simulink library "autolibshared"  (R2019b)
settings: Solver=ode45  StartTime=0.0  StopTime=10.0  RelTol=1e-3  EnableMultiTasking=on
undefined symbols (not defined in the file or in its folder): AccelCycle, aMode, DriveCycle, GearCycle, psi, x_o
libraries: autolibsharedcommon x20, $bdroot x7, autolibutils x2, autolibpowerinfoutils x1
(part 2 of 4)

== system autolibshared/Bicycle Model - Force Input ==
  WhlAngF : Inport  Unit=rad
  FxF : Inport  Port=2  Unit=N
  FxR : Inport  Port=3  Unit=N
  Terminator : Terminator
  Terminator1 : Terminator
  Vehicle Body 3DOF Single Track : $bdroot/Vehicle Body 3DOF Single Track  trackMode=Single (bicycle)  inputMode=External longitudinal forces  frontSteerMode=on  rearSteerMode=off  windMode=off  muMode=off  extFMode=off  extMMode=off  extXo=off  extpsio=off  extxdoto=off  extro=off  extYo=off  extTamb=off  extydoto=off  aMode=aMode  NF=NF  NR=NR  m=m  a=a  b=b  h=h  X_o=X_o  xdot_o=xdot_o  CalphaMode=off  sigmaMode=off  d=0  w=[1.4,1.4]  Cy_f=Cy_f  Cy_r=Cy_r  sigma_f=.1  sigma_r=.1  alpha_f_brk=[-.1 .1]  Cy_f_data=[-9e3 9e3]  alpha_r_brk=[-.1 .1]  Cy_r_data=[-9e3 9e3]  Y_o=Y_o  ydot_o=ydot_o  Izz=Izz  psi_o=psi_o  r_o=r_o  Af=Af  Cd=Cd  Cl=Cl  Cpm=Cpm  beta_w=beta_w  Cs=Cs  Cym=Cym  Pabs=Pabs  Tair=Tair  g=g  mu=mu  xdot_tol=xdot_tol  Fznom=Fznom  Fxtire_sat=Fxtire_sat  Fytire_sat=Fytire_sat  longOff=longOff  latOff=latOff  vertOff=vertOff  wrapAng=off
  Info : Outport  VectorParamsAs1DForOutWhenUnconnected=off
  xdot : Outport  Port=2  VectorParamsAs1DForOutWhenUnconnected=off
  ydot : Outport  Port=3  VectorParamsAs1DForOutWhenUnconnected=off
  psi : Outport  Port=4  VectorParamsAs1DForOutWhenUnconnected=off
  r : Outport  Port=5  VectorParamsAs1DForOutWhenUnconnected=off
  wires:
  Vehicle Body 3DOF Single Track/1 -> Info/1
  Vehicle Body 3DOF Single Track/4 -> psi/1
  WhlAngF/1 -> Vehicle Body 3DOF Single Track/1
  Vehicle Body 3DOF Single Track/2 -> xdot/1
  Vehicle Body 3DOF Single Track/3 -> ydot/1
  Vehicle Body 3DOF Single Track/5 -> r/1
  Vehicle Body 3DOF Single Track/6 -> Terminator1/1
  Vehicle Body 3DOF Single Track/7 -> Terminator/1
  FxF/1 -> Vehicle Body 3DOF Single Track/2
  FxR/1 -> Vehicle Body 3DOF Single Track/3

== system autolibshared/Bicycle Model - Velocity Input ==
  WhlAngF : Inport  Unit=rad
  xdotin : Inport  Port=2  Unit=m/s
  Terminator : Terminator
  Terminator1 : Terminator
  Vehicle Body 3DOF Single Track : $bdroot/Vehicle Body 3DOF Single Track  trackMode=Single (bicycle)  inputMode=External longitudinal velocity  frontSteerMode=on  rearSteerMode=off  windMode=off  muMode=off  extFMode=off  extMMode=off  extXo=off  extpsio=off  extxdoto=off  extro=off  extYo=off  extTamb=off  extydoto=off  aMode=aMode  NF=NF  NR=NR  m=m  a=a  b=b  h=h  X_o=X_o  xdot_o=xdot_o  CalphaMode=off  sigmaMode=off  d=0  w=[1.4,1.4]  Cy_f=Cy_f  Cy_r=Cy_r  sigma_f=.1  sigma_r=.1  alpha_f_brk=[-.1 .1]  Cy_f_data=[-9e3 9e3]  alpha_r_brk=[-.1 .1]  Cy_r_data=[-9e3 9e3]  Y_o=Y_o  ydot_o=ydot_o  Izz=Izz  psi_o=psi_o  r_o=r_o  Af=Af  Cd=Cd  Cl=Cl  Cpm=Cpm  beta_w=beta_w  Cs=Cs  Cym=Cym  Pabs=Pabs  Tair=Tair  g=g  mu=mu  xdot_tol=xdot_tol  Fznom=Fznom  Fxtire_sat=Fxtire_sat  Fytire_sat=Fytire_sat  longOff=longOff  latOff=latOff  vertOff=vertOff  wrapAng=off
  Info : Outport  VectorParamsAs1DForOutWhenUnconnected=off
  xdot : Outport  Port=2  VectorParamsAs1DForOutWhenUnconnected=off
  ydot : Outport  Port=3  VectorParamsAs1DForOutWhenUnconnected=off
  psi : Outport  Port=4  VectorParamsAs1DForOutWhenUnconnected=off
  r : Outport  Port=5  VectorParamsAs1DForOutWhenUnconnected=off
  wires:
  Vehicle Body 3DOF Single Track/7 -> Terminator/1
  xdotin/1 -> Vehicle Body 3DOF Single Track/2
  Vehicle Body 3DOF Single Track/6 -> Terminator1/1
  Vehicle Body 3DOF Single Track/5 -> r/1
  Vehicle Body 3DOF Single Track/3 -> ydot/1
  Vehicle Body 3DOF Single Track/2 -> xdot/1
  WhlAngF/1 -> Vehicle Body 3DOF Single Track/1
  Vehicle Body 3DOF Single Track/4 -> psi/1
  Vehicle Body 3DOF Single Track/1 -> Info/1

== system autolibshared/Drive Cycle Source ==
  Gear : Terminator
  Reference Accel : Terminator
  UnitConversion : UnitConversion
  timing mode : Subsystem  VariantControlMode=Label  Variant=on  LabelModeActiveChoice=1
  Reference Speed : Outport  Unit=m/s  VectorParamsAs1DForOutWhenUnconnected=off
  wires:
  timing mode/3(Gear) -> Gear/1
  UnitConversion/1 -> Reference Speed/1
  timing mode/1(Spd) -> UnitConversion/1
  timing mode/2(Acc) -> Reference Accel/1

== system autolibshared/Longitudinal Driver ==
  VelRef : Inport  Unit=m/s
  VelFdbk : Inport  Port=2  Unit=m/s
  Grade : Inport  Port=3
  ExtGear Ground : Ground
  Gear Terminator : Terminator
  Longitudinal Driver : autolibsharedcommon/Longitudinal Driver  cntrlType=PI  shftType=None  vnom=vnom  Kp=Kp  Ki=Ki  Kaw=Kaw  Kff=Kff  Kg=Kg  tauerr=tauerr  tShift=tShift  tRev=tRev  tPark=tPark  pdlVec=pdlVec  upShftTbl=upShftTbl  dwnShftTbl=dwnShftTbl  GearInit=GearInit  tClutch=tClutch  VehVelVec=VehVelVec  KffVec=KffVec  KiVec=KiVec  KpVec=KpVec  KgVec=KgVec  m=m  Kpt=Kpt  Lvv=L  g=g  UpGearVec=UpGearVec  DownGearVec=DownGearVec  aMode=aMode  errUnit=m/s  aR=aR  bR=bR  cR=cR  tauPt=tauPt
      settings: SourceProductName=Powertrain Blockset  SourceProductBaseCode=PW
  Info : Outport  InitialOutput=0  VectorParamsAs1DForOutWhenUnconnected=off
  AccelCmd : Outport  Port=2  VectorParamsAs1DForOutWhenUnconnected=off
  DecelCmd : Outport  Port=3  VectorParamsAs1DForOutWhenUnconnected=off
  wires:
  VelRef/1 -> Longitudinal Driver/1
  VelFdbk/1 -> Longitudinal Driver/2
  Longitudinal Driver/1 -> Info/1
  Longitudinal Driver/2 -> AccelCmd/1
  Longitudinal Driver/3 -> DecelCmd/1
  Longitudinal Driver/4 -> Gear Terminator/1
  ExtGear Ground/1 -> Longitudinal Driver/4
  Grade/1 -> Longitudinal Driver/3

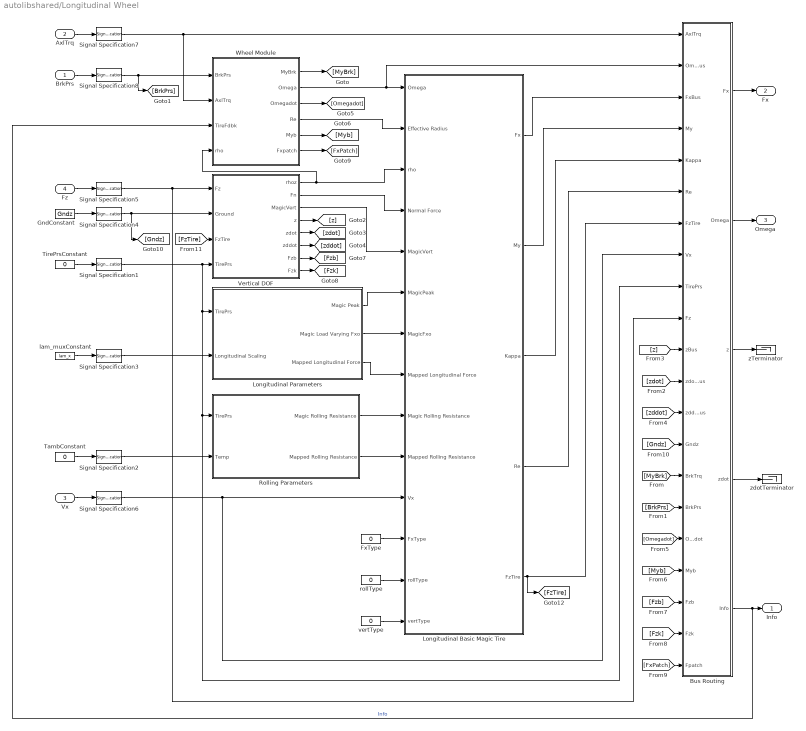
== system autolibshared/Longitudinal Wheel ==
  BrkPrs : Inport
  AxlTrq : Inport  Port=2
  Vx : Inport  Port=3
  Fz : Inport  Port=4
  Bus Routing : Subsystem
  FxType : Constant  Value=0
  GndConstant : Constant  Value=Gndz
  Longitudinal Basic Magic Tire : Subsystem
  Longitudinal Parameters : Subsystem  VariantControlMode=Label  Variant=on  LabelModeActiveChoice=MagicFormulaconstantvalueFx
  Rolling Parameters : Subsystem  VariantControlMode=Label  Variant=on  LabelModeActiveChoice=None
  Signal Specification1 : SignalSpecification  Unit=Pa
  Signal Specification2 : SignalSpecification  Unit=K
  Signal Specification3 : SignalSpecification  Unit=1
  Signal Specification4 : SignalSpecification  Unit=m
  Signal Specification5 : SignalSpecification  Unit=N
  Signal Specification6 : SignalSpecification  Unit=m/s
  Signal Specification7 : SignalSpecification  Unit=N*m
  Signal Specification8 : SignalSpecification  Unit=Pa
  TambConstant : Constant  Value=0
  TirePrsConstant : Constant  Value=0
  Vertical DOF : Subsystem  VariantControlMode=Label  Variant=on  LabelModeActiveChoice=None
  Wheel Module : Subsystem  mask(Wheel Module){aMode=aMode}
  lam_muxConstant : Constant  Value=lam_x
  rollType : Constant  Value=0
  vertType : Constant  Value=0
  zTerminator : Terminator
  zdotTerminator : Terminator
  Info : Outport  VectorParamsAs1DForOutWhenUnconnected=off
  Fx : Outport  Port=2  VectorParamsAs1DForOutWhenUnconnected=off
  Omega : Outport  Port=3  VectorParamsAs1DForOutWhenUnconnected=off
  wires:
  Bus Routing/1(Fx) -> Fx/1
  Bus Routing/5(Info) -> Info/1, Wheel Module/3(TireFdbk)  "Info"
  Bus Routing/2(Omega) -> Omega/1
  Bus Routing/3(z) -> zTerminator/1
  Bus Routing/4(zdot) -> zdotTerminator/1
  TirePrsConstant/1 -> Signal Specification1/1
  Signal Specification2/1 -> Rolling Parameters/2(Temp)
  [BrkPrs] -> Bus Routing/16(BrkPrs)
  Longitudinal Basic Magic Tire/4(Re) -> Bus Routing/6(Re)
  Rolling Parameters/2(Mapped Rolling Resistance) -> Longitudinal Basic Magic Tire/10(Mapped Rolling Resistance)
  Vertical DOF/5(zdot) -> [zdot]
  [zdot] -> Bus Routing/12(zdotBus)
  Longitudinal Basic Magic Tire/2(My) -> Bus Routing/4(My)
  FxType/1 -> Longitudinal Basic Magic Tire/12(FxType)
  Rolling Parameters/1(Magic Rolling Resistance) -> Longitudinal Basic Magic Tire/9(Magic Rolling Resistance)
  Vertical DOF/4(z) -> [z]
  Vertical DOF/3(MagicVert) -> Longitudinal Basic Magic Tire/5(MagicVert)
  Vertical DOF/2(Fn) -> Longitudinal Basic Magic Tire/4(Normal Force)
  rollType/1 -> Longitudinal Basic Magic Tire/13(rollType)
  Longitudinal Parameters/3(Mapped Longitudinal Force) -> Longitudinal Basic Magic Tire/8(Mapped Longitudinal Force)
  Fz/1 -> Signal Specification5/1
  Longitudinal Basic Magic Tire/5(FzTire) -> Bus Routing/7(FzTire), [FzTire]
  Vx/1 -> Signal Specification6/1
  [z] -> Bus Routing/11(zBus)
  Longitudinal Parameters/2(Magic Load Varying Fxo) -> Longitudinal Basic Magic Tire/7(MagicFxo)
  [MyBrk] -> Bus Routing/15(BrkTrq)
  vertType/1 -> Longitudinal Basic Magic Tire/14(vertType)
  AxlTrq/1 -> Signal Specification7/1
  Longitudinal Parameters/1(Magic Peak) -> Longitudinal Basic Magic Tire/6(MagicPeak)
  Vertical DOF/1(rhoz) -> Wheel Module/4(rho), Longitudinal Basic Magic Tire/3(rho)
  Longitudinal Basic Magic Tire/3(Kappa) -> Bus Routing/5(Kappa)
  Longitudinal Basic Magic Tire/1(Fx) -> Bus Routing/3(FxBus)
  Wheel Module/1(MyBrk) -> [MyBrk]
  Wheel Module/2(Omega) -> Bus Routing/2(OmegaBus), Longitudinal Basic Magic Tire/1(Omega)
  Signal Specification1/1 -> Bus Routing/9(TirePrs), Rolling Parameters/1(TirePrs), Longitudinal Parameters/1(TirePrs), Vertical DOF/4(TirePrs)
  Signal Specification3/1 -> Longitudinal Parameters/2(Longitudinal Scaling)
  Signal Specification4/1 -> Vertical DOF/2(Ground), [Gndz]
  Signal Specification5/1 -> Vertical DOF/1(Fz), Bus Routing/10(Fz)
  Signal Specification6/1 -> Longitudinal Basic Magic Tire/11(Vx), Bus Routing/8(Vx)
  Signal Specification7/1 -> Bus Routing/1(AxlTrq), Wheel Module/2(AxlTrq)
  Signal Specification8/1 -> [BrkPrs], Wheel Module/1(BrkPrs)
  lam_muxConstant/1 -> Signal Specification3/1
  TambConstant/1 -> Signal Specification2/1
  Wheel Module/4(Re) -> Longitudinal Basic Magic Tire/2(Effective Radius)
  Vertical DOF/6(zddot) -> [zddot]
  [zddot] -> Bus Routing/13(zddotBus)
  Wheel Module/3(Omegadot) -> [Omegadot]
  [Omegadot] -> Bus Routing/17(Omegadot)
  Wheel Module/5(Myb) -> [Myb]
  [Myb] -> Bus Routing/18(Myb)
  Vertical DOF/8(Fzk) -> [Fzk]
  Vertical DOF/7(Fzb) -> [Fzb]
  [Fzb] -> Bus Routing/19(Fzb)
  [Fzk] -> Bus Routing/20(Fzk)
  Wheel Module/6(Fxpatch) -> [FxPatch]
  [FxPatch] -> Bus Routing/21(Fpatch)
  GndConstant/1 -> Signal Specification4/1
  [Gndz] -> Bus Routing/14(Gndz)
  [FzTire] -> Vertical DOF/3(FzTire)
  BrkPrs/1 -> Signal Specification8/1

== system autolibshared/Vehicle Body 1DOF Longitudinal ==
  FwF : Inport
  FwR : Inport  Port=2
  Grade : Inport  Port=3
  WindX : Inport  Port=4
  AirTempConstant : Constant  Value=T
  FExtConstant : Constant  Value=[0,0,0]
  MExtConstant : Constant  Value=[0,0,0]
  Vehicle Body 1 DOF : autolibsharedcommon/Vehicle Body 1 DOF  VariantControl=SL1dof  m=m  NF=NF  NR=NR  a=a  b=b  h=h  Af=Af  Cd=Cd  Cl=Cl  Cpm=Cpm  T=T  Pabs=Pabs  xdot_o=xdot_o  g=g  aMode=aMode
      settings: SourceProductName=Powertrain Blockset  SourceProductBaseCode=PW
  Info : Outport  VectorParamsAs1DForOutWhenUnconnected=off
  xdot : Outport  Port=2  PortDimensions=1  VectorParamsAs1DForOutWhenUnconnected=off
  FzF : Outport  Port=3  PortDimensions=1  VectorParamsAs1DForOutWhenUnconnected=off
  FzR : Outport  Port=4  PortDimensions=1  VectorParamsAs1DForOutWhenUnconnected=off
  wires:
  FwF/1 -> Vehicle Body 1 DOF/1
  FwR/1 -> Vehicle Body 1 DOF/2
  Grade/1 -> Vehicle Body 1 DOF/3
  WindX/1 -> Vehicle Body 1 DOF/4
  Vehicle Body 1 DOF/1 -> Info/1
  Vehicle Body 1 DOF/2 -> xdot/1
  Vehicle Body 1 DOF/3 -> FzF/1
  Vehicle Body 1 DOF/4 -> FzR/1
  FExtConstant/1 -> Vehicle Body 1 DOF/5
  MExtConstant/1 -> Vehicle Body 1 DOF/6
  AirTempConstant/1 -> Vehicle Body 1 DOF/7

== system autolibshared/Vehicle Body 3DOF Longitudinal ==
  FwF : Inport
  FwR : Inport  Port=2
  Grade : Inport  Port=3
  WindXYZ : Inport  Port=4
  AirTempConstant : Constant  Value=T
  FExtConstant : Constant  Value=[0,0,0]
  MExtConstant : Constant  Value=[0,0,0]
  Vehicle Body 3 DOF Grade Input : autolibsharedcommon/Vehicle Body 3 DOF Grade Input  VariantControl=SL  NF=NF  NR=NR  m=m  a=a  b=b  h=h  Cd=Cd  Af=Af  x_o=x_o  xdot_o=xdot_o  Cl=Cl  z_o=z_o  zdot_o=zdot_o  Iyy=Iyy  Cpm=Cpm  theta_o=theta_o  q_o=q_o  FskF=FskF  dzsF=dzsF  FsbF=FsbF  dzdotsF=dzdotsF  FskR=FskR  dzsR=dzsR  FsbR=FsbR  dzdotsR=dzdotsR  Pabs=Pabs  T=T  g=g  aMode=aMode
      settings: SourceProductName=Powertrain Blockset  SourceProductBaseCode=PW
  Info : Outport  VectorParamsAs1DForOutWhenUnconnected=off
  xdot : Outport  Port=2  VectorParamsAs1DForOutWhenUnconnected=off
  FzF : Outport  Port=3  VectorParamsAs1DForOutWhenUnconnected=off
  FzR : Outport  Port=4  VectorParamsAs1DForOutWhenUnconnected=off
  wires:
  FwF/1 -> Vehicle Body 3 DOF Grade Input/1
  FwR/1 -> Vehicle Body 3 DOF Grade Input/2
  Grade/1 -> Vehicle Body 3 DOF Grade Input/3
  AirTempConstant/1 -> Vehicle Body 3 DOF Grade Input/7
  WindXYZ/1 -> Vehicle Body 3 DOF Grade Input/4
  Vehicle Body 3 DOF Grade Input/3 -> FzF/1
  Vehicle Body 3 DOF Grade Input/4 -> FzR/1
  Vehicle Body 3 DOF Grade Input/1 -> Info/1
  Vehicle Body 3 DOF Grade Input/2 -> xdot/1
  FExtConstant/1 -> Vehicle Body 3 DOF Grade Input/5
  MExtConstant/1 -> Vehicle Body 3 DOF Grade Input/6

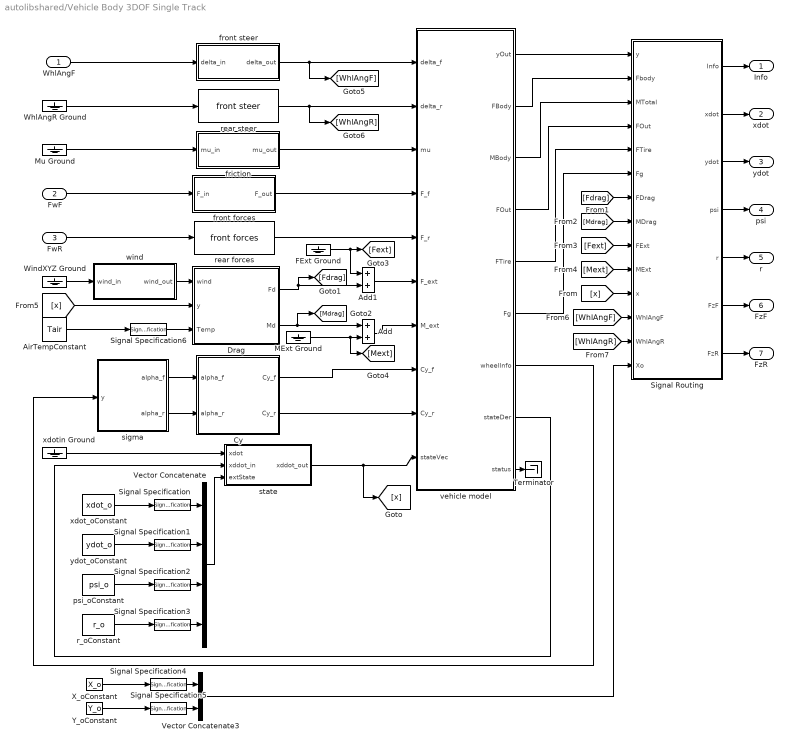
== system autolibshared/Vehicle Body 3DOF Single Track ==
  WhlAngF : Inport
  FwF : Inport  Port=2
  FwR : Inport  Port=3
  Add : Sum
  Add1 : Sum
  AirTempConstant : Constant  Value=Tair
  Cy : Subsystem  VariantControlMode=Label  Variant=on  LabelModeActiveChoice=2
  Drag : Subsystem
  FExt Ground : Ground
  MExt Ground : Ground
  Mu Ground : Ground
  Signal Routing : Subsystem  VariantControlMode=Label  Variant=on  LabelModeActiveChoice=1
  Signal Specification : SignalSpecification  Unit=m/s
  Signal Specification1 : SignalSpecification  Unit=m/s
  Signal Specification2 : SignalSpecification  Unit=rad
  Signal Specification3 : SignalSpecification  Unit=rad/s
  Signal Specification4 : SignalSpecification  Unit=m
  Signal Specification5 : SignalSpecification  Unit=m
  Signal Specification6 : SignalSpecification  Unit=K
  Terminator : Terminator
  Vector Concatenate : Concatenate  NumInputs=4
  Vector Concatenate3 : Concatenate
  WhlAngR Ground : Ground
  WindXYZ Ground : Ground
  X_oConstant : Constant  Value=X_o
  Y_oConstant : Constant  Value=Y_o
  friction : Subsystem  VariantControlMode=Label  Variant=on  LabelModeActiveChoice=2
  front forces : Subsystem  VariantControlMode=Label  Variant=on  LabelModeActiveChoice=4
  front steer : Subsystem  VariantControlMode=Label  Variant=on  LabelModeActiveChoice=3
  psi_oConstant : Constant  Value=psi_o
  r_oConstant : Constant  Value=r_o
  rear forces : $bdroot/Vehicle Body 3DOF Single Track/front forces  SystemSampleTime=-1  LabelModeActiveChoice=4  Latency=0  AutoFrameSizeCalculation=off
  rear steer : $bdroot/Vehicle Body 3DOF Single Track/front steer  SystemSampleTime=-1  LabelModeActiveChoice=2  Latency=0  AutoFrameSizeCalculation=off
  sigma : Subsystem  VariantControlMode=Label  Variant=on  LabelModeActiveChoice=2
  state : Subsystem  VariantControlMode=Label  Variant=on  LabelModeActiveChoice=0
  vehicle model : MATLAB Function  TreatAsAtomicUnit=on
  wind : Subsystem  VariantControlMode=Label  Variant=on  LabelModeActiveChoice=0
  xdot_oConstant : Constant  Value=xdot_o
  xdotin Ground : Ground
  ydot_oConstant : Constant  Value=ydot_o
  Info : Outport  VectorParamsAs1DForOutWhenUnconnected=off
  xdot : Outport  Port=2  VectorParamsAs1DForOutWhenUnconnected=off
  ydot : Outport  Port=3  VectorParamsAs1DForOutWhenUnconnected=off
  psi : Outport  Port=4  VectorParamsAs1DForOutWhenUnconnected=off
  r : Outport  Port=5  VectorParamsAs1DForOutWhenUnconnected=off
  FzF : Outport  Port=6  VectorParamsAs1DForOutWhenUnconnected=off
  FzR : Outport  Port=7  VectorParamsAs1DForOutWhenUnconnected=off
  wires:
  Add1/1 -> vehicle model/6(F_ext)
  Add/1 -> vehicle model/7(M_ext)
  vehicle model/3(MBody) -> Signal Routing/3(MTotal)
  vehicle model/2(FBody) -> Signal Routing/2(Fbody)
  [Mext] -> Signal Routing/10(MExt)
  [Mdrag] -> Signal Routing/8(MDrag)
  [Fdrag] -> Signal Routing/7(FDrag)
  [Fext] -> Signal Routing/9(FExt)
  vehicle model/6(Fg) -> Signal Routing/6(Fg)
  vehicle model/5(FTire) -> Signal Routing/5(FTire)
  vehicle model/9(status) -> Terminator/1
  [x] -> Signal Routing/11(x)
  state/1(xddot_out) -> vehicle model/10(stateVec), [x]
  vehicle model/4(FOut) -> Signal Routing/4(FOut)
  Signal Routing/2(xdot) -> xdot/1
  Signal Routing/7(FzR) -> FzR/1
  Signal Routing/6(FzF) -> FzF/1
  Signal Routing/5(r) -> r/1
  Signal Routing/3(ydot) -> ydot/1
  vehicle model/1(yOut) -> Signal Routing/1(y)
  vehicle model/8(stateDer) -> state/2(xddot_in)
  friction/1(mu_out) -> vehicle model/3(mu)
  Cy/1(Cy_f) -> vehicle model/8(Cy_f)
  Cy/2(Cy_r) -> vehicle model/9(Cy_r)
  front steer/1(delta_out) -> [WhlAngF], vehicle model/1(delta_f)
  rear steer/1 -> [WhlAngR], vehicle model/2(delta_r)
  sigma/1(alpha_f) -> Cy/1(alpha_f)
  sigma/2(alpha_r) -> Cy/2(alpha_r)
  Signal Routing/1(Info) -> Info/1
  vehicle model/7(wheelInfo) -> sigma/1(y)
  front forces/1(F_out) -> vehicle model/4(F_f)
  rear forces/1 -> vehicle model/5(F_r)
  Drag/2(Md) -> [Mdrag], Add/1
  wind/1(wind_out) -> Drag/1(wind)
  Drag/1(Fd) -> Add1/2, [Fdrag]
  WindXYZ Ground/1 -> wind/1(wind_in)
  [x] -> Drag/2(y)
  WhlAngF/1 -> front steer/1(delta_in)
  WhlAngR Ground/1 -> rear steer/1
  Mu Ground/1 -> friction/1(mu_in)
  Signal Routing/4(psi) -> psi/1
  [WhlAngF] -> Signal Routing/12(WhlAngF)
  [WhlAngR] -> Signal Routing/13(WhlAngR)
  Vector Concatenate/1 -> state/3(extState)
  xdot_oConstant/1 -> Signal Specification/1
  Signal Specification/1 -> Vector Concatenate/1
  ydot_oConstant/1 -> Signal Specification1/1
  Signal Specification1/1 -> Vector Concatenate/2
  r_oConstant/1 -> Signal Specification3/1
  psi_oConstant/1 -> Signal Specification2/1
  Signal Specification3/1 -> Vector Concatenate/4
  Signal Specification2/1 -> Vector Concatenate/3
  Vector Concatenate3/1 -> Signal Routing/14(Xo)
  X_oConstant/1 -> Signal Specification4/1
  Signal Specification4/1 -> Vector Concatenate3/1
  Y_oConstant/1 -> Signal Specification5/1
  Signal Specification5/1 -> Vector Concatenate3/2
  Signal Specification6/1 -> Drag/3(Temp)
  AirTempConstant/1 -> Signal Specification6/1
  xdotin Ground/1 -> state/1(xdot)
  FwF/1 -> front forces/1(F_in)
  FwR/1 -> rear forces/1
  MExt Ground/1 -> [Mext], Add/2
  FExt Ground/1 -> Add1/1, [Fext]

== system autolibshared/Vehicle Body Total Road Load ==
  ForceTot : Inport
  Grade : Inport  Port=2
  Vehicle Body Total Road Load : autolibsharedcommon/Vehicle Body Total Road Load  VariantControl=SL1dof  m=m  a=a  b=b  c=c  xdot_o=xdot_o  g=g  x_o=x_o  aMode=aMode
      settings: SourceProductName=Powertrain Blockset  SourceProductBaseCode=PW
  Info : Outport  VectorParamsAs1DForOutWhenUnconnected=off
  xdot : Outport  Port=2  VectorParamsAs1DForOutWhenUnconnected=off
  wires:
  Grade/1 -> Vehicle Body Total Road Load/2
  ForceTot/1 -> Vehicle Body Total Road Load/1
  Vehicle Body Total Road Load/1 -> Info/1
  Vehicle Body Total Road Load/2 -> xdot/1

== system autolibshared/Drive Cycle Source/timing mode ==
  note: 1) Add Subsystem or Model blocks as valid variant choices.
      | 2) You cannot connect blocks at this level. At simulation, connectivity is automatically
      | determined, based on the active variant and port name matching.
  Continuous : Subsystem  VariantControl=1
  Discrete : Subsystem  VariantControl=2
  Spd : Outport  VectorParamsAs1DForOutWhenUnconnected=off
  Acc : Outport  Port=2  VectorParamsAs1DForOutWhenUnconnected=off
  Gear : Outport  Port=3  VectorParamsAs1DForOutWhenUnconnected=off

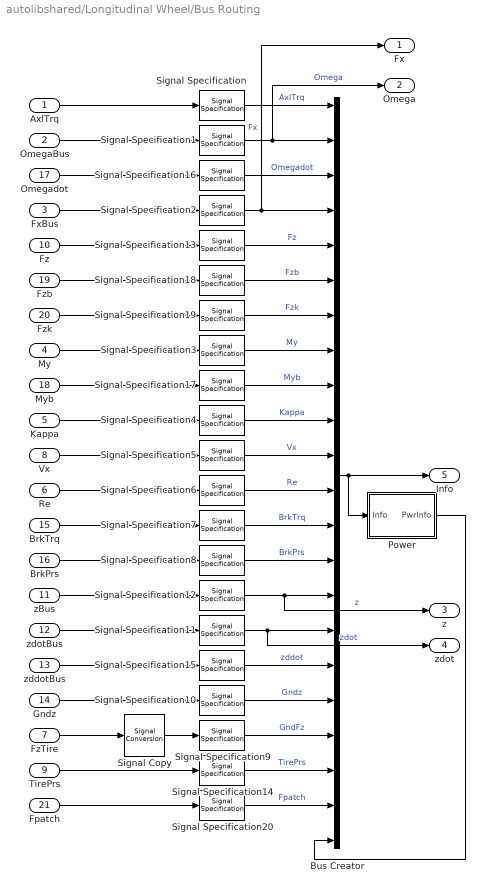
== system autolibshared/Longitudinal Wheel/Bus Routing ==
  AxlTrq : Inport
  OmegaBus : Inport  Port=2
  FxBus : Inport  Port=3
  My : Inport  Port=4
  Kappa : Inport  Port=5
  Re : Inport  Port=6
  FzTire : Inport  Port=7
  Vx : Inport  Port=8
  TirePrs : Inport  Port=9
  Fz : Inport  Port=10
  zBus : Inport  Port=11
  zdotBus : Inport  Port=12
  zddotBus : Inport  Port=13
  Gndz : Inport  Port=14
  BrkTrq : Inport  Port=15
  BrkPrs : Inport  Port=16
  Omegadot : Inport  Port=17
  Myb : Inport  Port=18
  Fzb : Inport  Port=19
  Fzk : Inport  Port=20
  Fpatch : Inport  Port=21
  Bus Creator : BusCreator  Inputs=22
  Power : Subsystem
  Signal Copy : SignalConversion  OverrideOpt=off
  Signal Specification{,3,7,17} (4 alike) : SignalSpecification  Unit=N*m
  Signal Specification1 : SignalSpecification  Unit=rad/s
  Signal Specification10 : SignalSpecification  Unit=m
  Signal Specification11 : SignalSpecification  Unit=m/s
  Signal Specification12 : SignalSpecification  Unit=m
  Signal Specification{2,9,13,18..20} (6 alike) : SignalSpecification  Unit=N
  Signal Specification14 : SignalSpecification  Unit=Pa
  Signal Specification15 : SignalSpecification  Unit=m/s^2
  Signal Specification16 : SignalSpecification  Unit=rad/s^2
  Signal Specification4 : SignalSpecification  Unit=1
  Signal Specification5 : SignalSpecification  Unit=m/s
  Signal Specification6 : SignalSpecification  Unit=m
  Signal Specification8 : SignalSpecification  Unit=Pa
  Fx : Outport  Unit=N  VectorParamsAs1DForOutWhenUnconnected=off
  Omega : Outport  Port=2  Unit=rad/s  VectorParamsAs1DForOutWhenUnconnected=off
  z : Outport  Port=3  Unit=m  VectorParamsAs1DForOutWhenUnconnected=off
  zdot : Outport  Port=4  Unit=m/s  VectorParamsAs1DForOutWhenUnconnected=off
  Info : Outport  Port=5  VectorParamsAs1DForOutWhenUnconnected=off
  wires:
  Signal Specification14/1 -> Bus Creator/20  "TirePrs"
  TirePrs/1 -> Signal Specification14/1
  Re/1 -> Signal Specification6/1
  Fz/1 -> Signal Specification13/1
  Signal Specification13/1 -> Bus Creator/5  "Fz"
  Signal Specification12/1 -> z/1, Bus Creator/15  "z"
  Signal Specification11/1 -> zdot/1, Bus Creator/16  "zdot"
  zdotBus/1 -> Signal Specification11/1
  FzTire/1 -> Signal Copy/1
  Signal Specification9/1 -> Bus Creator/19  "GndFz"
  zBus/1 -> Signal Specification12/1
  Signal Specification5/1 -> Bus Creator/11  "Vx"
  Signal Specification2/1 -> Bus Creator/4, Fx/1  "Fx"
  BrkTrq/1 -> Signal Specification7/1
  Signal Specification/1 -> Bus Creator/1  "AxlTrq"
  Signal Specification3/1 -> Bus Creator/8  "My"
  Signal Specification1/1 -> Bus Creator/2, Omega/1  "Omega"
  BrkPrs/1 -> Signal Specification8/1
  Signal Specification4/1 -> Bus Creator/10  "Kappa"
  Signal Specification8/1 -> Bus Creator/14  "BrkPrs"
  Kappa/1 -> Signal Specification4/1
  My/1 -> Signal Specification3/1
  Signal Specification6/1 -> Bus Creator/12  "Re"
  Signal Specification7/1 -> Bus Creator/13  "BrkTrq"
  Bus Creator/1 -> Info/1, Power/1(Info)
  Signal Specification10/1 -> Bus Creator/18  "Gndz"
  FxBus/1 -> Signal Specification2/1
  AxlTrq/1 -> Signal Specification/1
  Gndz/1 -> Signal Specification10/1
  Vx/1 -> Signal Specification5/1
  Signal Specification15/1 -> Bus Creator/17  "zddot"
  zddotBus/1 -> Signal Specification15/1
  Omegadot/1 -> Signal Specification16/1
  Signal Specification16/1 -> Bus Creator/3  "Omegadot"
  Myb/1 -> Signal Specification17/1
  Signal Specification17/1 -> Bus Creator/9  "Myb"
  Fzb/1 -> Signal Specification18/1
  Fzk/1 -> Signal Specification19/1
  Signal Specification18/1 -> Bus Creator/6  "Fzb"
  Signal Specification19/1 -> Bus Creator/7  "Fzk"
  Fpatch/1 -> Signal Specification20/1
  Signal Specification20/1 -> Bus Creator/21  "Fpatch"
  Power/1(PwrInfo) -> Bus Creator/22
  Signal Copy/1 -> Signal Specification9/1
  OmegaBus/1 -> Signal Specification1/1

== system autolibshared/Longitudinal Wheel/Longitudinal Basic Magic Tire ==
  Omega : Inport
  Effective Radius : Inport  Port=2
  rho : Inport  Port=3
  Normal Force : Inport  Port=4
  MagicVert : Inport  Port=5
  MagicPeak : Inport  Port=6
  MagicFxo : Inport  Port=7
  Mapped Longitudinal Force : Inport  Port=8
  Magic Rolling Resistance : Inport  Port=9
  Mapped Rolling Resistance : Inport  Port=10
  Vx : Inport  Port=11
  FxType : Inport  Port=12
  rollType : Inport  Port=13
  vertType : Inport  Port=14
  Bus Selector1 : BusSelector  OutputSignals=VxMy,FzMy,MyMap
  Bus Selector2 : BusSelector  OutputSignals=kappaFx,FzFx,FxMap
  Bus to Vector{,1..3} (4 alike) : BusToVector
  Simple Magic Tire : MATLAB Function
  Fx : Outport  VectorParamsAs1DForOutWhenUnconnected=off
  My : Outport  Port=2  VectorParamsAs1DForOutWhenUnconnected=off
  Kappa : Outport  Port=3  VectorParamsAs1DForOutWhenUnconnected=off
  Re : Outport  Port=4  VectorParamsAs1DForOutWhenUnconnected=off
  FzTire : Outport  Port=5  VectorParamsAs1DForOutWhenUnconnected=off
  wires:
  Simple Magic Tire/4(Re) -> Re/1
  Bus to Vector3/1 -> Simple Magic Tire/15(MagicVert)
  MagicVert/1 -> Bus to Vector3/1
  Simple Magic Tire/5(FzTire) -> FzTire/1
  rho/1 -> Simple Magic Tire/14(rho)
  vertType/1 -> Simple Magic Tire/18(vertType)
  Bus to Vector2/1 -> Simple Magic Tire/5(MagicPeak)
  Bus to Vector1/1 -> Simple Magic Tire/6(MagicFxo)
  Bus to Vector/1 -> Simple Magic Tire/10(RollRes)
  MagicFxo/1 -> Bus to Vector1/1
  MagicPeak/1 -> Bus to Vector2/1
  Bus Selector2/3 -> Simple Magic Tire/9(FxMap)  "<FxMap>"
  Bus Selector2/2 -> Simple Magic Tire/8(FzFx)  "<FzFx>"
  Bus Selector2/1 -> Simple Magic Tire/7(kappaFx)  "<kappaFx>"
  Mapped Longitudinal Force/1 -> Bus Selector2/1
  Bus Selector1/3 -> Simple Magic Tire/13(MyMap)  "<MyMap>"
  Bus Selector1/2 -> Simple Magic Tire/12(FzMy)  "<FzMy>"
  Bus Selector1/1 -> Simple Magic Tire/11(VxMy)  "<VxMy>"
  Mapped Rolling Resistance/1 -> Bus Selector1/1
  rollType/1 -> Simple Magic Tire/17(rollingType)
  FxType/1 -> Simple Magic Tire/16(FxType)
  Magic Rolling Resistance/1 -> Bus to Vector/1
  Vx/1 -> Simple Magic Tire/4(Vx)
  Omega/1 -> Simple Magic Tire/3(Omega)
  Simple Magic Tire/1(Fx) -> Fx/1
  Normal Force/1 -> Simple Magic Tire/2(Fz)
  Simple Magic Tire/3(Kappa) -> Kappa/1
  Effective Radius/1 -> Simple Magic Tire/1(ReNom)
  Simple Magic Tire/2(My) -> My/1

== system autolibshared/Longitudinal Wheel/Longitudinal Parameters ==
  note: 1) Add Subsystem or Model blocks as valid variant choices.
      | 2) You cannot connect blocks at this level. At simulation, connectivity is automatically
      | determined, based on the active variant and port name matching.
  TirePrs : Inport
  Longitudinal Scaling : Inport  Port=2
  Magic Formula Load Varying : Subsystem  VariantControl=MagicFormulapurelongitudinalslipFx
  Magic Formula Peak Value : Subsystem  VariantControl=MagicFormulaconstantvalueFx
  Mapped Force : Subsystem  VariantControl=Mappedforce
  Magic Peak : Outport  VectorParamsAs1DForOutWhenUnconnected=off
  Magic Load Varying Fxo : Outport  Port=2  VectorParamsAs1DForOutWhenUnconnected=off
  Mapped Longitudinal Force : Outport  Port=3  VectorParamsAs1DForOutWhenUnconnected=off

== system autolibshared/Longitudinal Wheel/Rolling Parameters ==
  note: 1) Add Subsystem or Model blocks as valid variant choices.
      | 2) You cannot connect blocks at this level. At simulation, connectivity is automatically
      | determined, based on the active variant and port name matching.
  TirePrs : Inport  Unit=Pa
  Temp : Inport  Port=2  Unit=K
  ISO : Subsystem  VariantControl=ISO
  Magic : Subsystem  VariantControl=MagicFormula
  Mapped : Subsystem  VariantControl=Mappedtorque
  None : Subsystem  VariantControl=None
  Simple : Subsystem  VariantControl=Simple
  Magic Rolling Resistance : Outport  VectorParamsAs1DForOutWhenUnconnected=off
  Mapped Rolling Resistance : Outport  Port=2  VectorParamsAs1DForOutWhenUnconnected=off

== system autolibshared/Longitudinal Wheel/Vertical DOF ==
  note: 1) Add Subsystem or Model blocks as valid variant choices.
      | 2) You cannot connect blocks at this level. At simulation, connectivity is automatically
      | determined, based on the active variant and port name matching.
  Fz : Inport
  Ground : Inport  Port=2
  FzTire : Inport  Port=3
  TirePrs : Inport  Port=4
  Magic Vertical DOF : Subsystem  VariantControl=Magic
  Mapped Vertical DOF : Subsystem  VariantControl=Mapped
  None : Subsystem  VariantControl=None
  rhoz : Outport  VectorParamsAs1DForOutWhenUnconnected=off
  Fn : Outport  Port=2  VectorParamsAs1DForOutWhenUnconnected=off
  MagicVert : Outport  Port=3  VectorParamsAs1DForOutWhenUnconnected=off
  z : Outport  Port=4  VectorParamsAs1DForOutWhenUnconnected=off
  zdot : Outport  Port=5  VectorParamsAs1DForOutWhenUnconnected=off
  zddot : Outport  Port=6  VectorParamsAs1DForOutWhenUnconnected=off
  Fzb : Outport  Port=7  VectorParamsAs1DForOutWhenUnconnected=off
  Fzk : Outport  Port=8  VectorParamsAs1DForOutWhenUnconnected=off

== system autolibshared/Longitudinal Wheel/Wheel Module ==
  BrkPrs : Inport
  AxlTrq : Inport  Port=2
  TireFdbk : Inport  Port=3
  rho : Inport  Port=4
  Add1 : Sum  Inputs=+-
  Add2 : Sum
  Brakes : Subsystem  VariantControlMode=Label  Variant=on  LabelModeActiveChoice=Disk
  Bus Selector1 : BusSelector  OutputSignals=Fx,My
  Clutch : Stateflow chart  TreatAsAtomicUnit=on  mask{OmegaTol=pi/30}
  Constant9 : Constant  Value=Re
  Friction Model : Subsystem
  Sign convention : Gain  Gain=-1
  Terminator2 : Terminator
  relaxation : autolibsharedcommon/Longitudinal Wheel/wheel dynamics/relaxation  aMode=aMode
      settings: SourceProductName=Powertrain Blockset  SourceProductBaseCode=PW
  MyBrk : Outport  VectorParamsAs1DForOutWhenUnconnected=off
  Omega : Outport  Port=2  VectorParamsAs1DForOutWhenUnconnected=off
  Omegadot : Outport  Port=3  VectorParamsAs1DForOutWhenUnconnected=off
  Re : Outport  Port=4  VectorParamsAs1DForOutWhenUnconnected=off
  Myb : Outport  Port=5  VectorParamsAs1DForOutWhenUnconnected=off
  Fxpatch : Outport  Port=6  VectorParamsAs1DForOutWhenUnconnected=off
  wires:
  Add2/1 -> Re/1, relaxation/3
  Constant9/1 -> Add2/2
  rho/1 -> Add2/1
  AxlTrq/1 -> Add1/1
  Sign convention/1 -> Clutch/1(Tout)
  BrkPrs/1 -> Brakes/1(BrkPrs)
  relaxation/1 -> Add1/2
  Add1/1 -> Sign convention/1
  Bus Selector1/1 -> relaxation/1  "<Fx>"
  Bus Selector1/2 -> relaxation/2  "<My>"
  TireFdbk/1 -> Bus Selector1/1
  Clutch/2(Omegadot) -> Omegadot/1
  Clutch/3(Myb) -> Myb/1
  relaxation/2 -> Fxpatch/1
  Brakes/1(MyBrk) -> MyBrk/1, Friction Model/1(Brake torque)
  Clutch/1(Omega) -> Brakes/2(Omega), relaxation/4, Omega/1
  Friction Model/2(Tfmaxk) -> Clutch/3(Tfmaxk)
  Friction Model/1(Tfmaxs) -> Clutch/2(Tfmaxs)
  Clutch/4(ReactionTorque) -> Terminator2/1

== system autolibshared/Vehicle Body 3DOF Single Track/Cy ==
  note: 1) Add Subsystem or Model blocks as valid variant choices.
      | 2) You cannot connect blocks at this level. At simulation, connectivity is automatically
      | determined, based on the active variant and port name matching.
  alpha_f : Inport
  alpha_r : Inport  Port=2
  Cy const : Subsystem  VariantControl=0
  Cy const dual : Subsystem  VariantControl=2
  Cy table : Subsystem  VariantControl=1
  Cy table dual : Subsystem  VariantControl=3
  Cy_f : Outport  VectorParamsAs1DForOutWhenUnconnected=off
  Cy_r : Outport  Port=2  VectorParamsAs1DForOutWhenUnconnected=off

== system autolibshared/Vehicle Body 3DOF Single Track/Drag ==
  wind : Inport
  y : Inport  Port=2
  Temp : Inport  Port=3  Unit=K
  Demux : Demux  Outputs=3
  Drag Force : autolibsharedcommon/Vehicle Body 3dof/Drag Force  A=Af  beta_w=beta_w  Cd=Cd  Cs=Cs  Cl=Cl  Cpm=Cpm  Lcpm=a+b  Crm=beta_w.*0  Cym=Cym  R=287.058  Pabs=Pabs
      settings: SourceProductName=Powertrain Blockset  SourceProductBaseCode=PW
  Ground : Ground
  Selector2 : Selector  InputPortWidth=4  IndexOptions=Index vector (dialog)  Indices=[1:3]  OutputSizes=1
  Unary Minus : UnaryMinus
  Unary Minus1 : UnaryMinus
  Vector Concatenate1 : Concatenate  NumInputs=3
  inertial2body : Subsystem
  Fd : Outport  VectorParamsAs1DForOutWhenUnconnected=off
  Md : Outport  Port=2  VectorParamsAs1DForOutWhenUnconnected=off
  wires:
  Unary Minus1/1 -> Md/1
  Unary Minus/1 -> Fd/1
  Drag Force/1 -> Unary Minus/1
  y/1 -> Selector2/1
  Drag Force/2 -> Unary Minus1/1
  Selector2/1 -> Demux/1
  Vector Concatenate1/1 -> Drag Force/1
  Ground/1 -> Vector Concatenate1/3
  Demux/2 -> Vector Concatenate1/2
  Demux/1 -> Vector Concatenate1/1
  Demux/3 -> inertial2body/1(psi)
  wind/1 -> inertial2body/2(WindXYZ)
  inertial2body/1(Windxyz) -> Drag Force/2
  Temp/1 -> Drag Force/3

== system autolibshared/Vehicle Body 3DOF Single Track/Signal Routing ==
  note: 1) Add Subsystem or Model blocks as valid variant choices.
      | 2) You cannot connect blocks at this level. At simulation, connectivity is automatically
      | determined, based on the active variant and port name matching.
  y : Inport
  Fbody : Inport  Port=2  Unit=N
  MTotal : Inport  Port=3  Unit=N*m
  FOut : Inport  Port=4
  FTire : Inport  Port=5  Unit=N
  Fg : Inport  Port=6  Unit=N
  FDrag : Inport  Port=7  Unit=N
  MDrag : Inport  Port=8  Unit=N*m
  FExt : Inport  Port=9  Unit=N
  MExt : Inport  Port=10  Unit=N*m
  x : Inport  Port=11
  WhlAngF : Inport  Port=12
  WhlAngR : Inport  Port=13
  Xo : Inport  Port=14
  Signal Routing : Subsystem  VariantControl=0
  Signal Routing Dual : Subsystem  VariantControl=1
  Info : Outport  VectorParamsAs1DForOutWhenUnconnected=off
  xdot : Outport  Port=2  VectorParamsAs1DForOutWhenUnconnected=off
  ydot : Outport  Port=3  VectorParamsAs1DForOutWhenUnconnected=off
  psi : Outport  Port=4  VectorParamsAs1DForOutWhenUnconnected=off
  r : Outport  Port=5  VectorParamsAs1DForOutWhenUnconnected=off
  FzF : Outport  Port=6  VectorParamsAs1DForOutWhenUnconnected=off
  FzR : Outport  Port=7  VectorParamsAs1DForOutWhenUnconnected=off

== system autolibshared/Vehicle Body 3DOF Single Track/friction ==
  note: 1) Add Subsystem or Model blocks as valid variant choices.
      | 2) You cannot connect blocks at this level. At simulation, connectivity is automatically
      | determined, based on the active variant and port name matching.
  mu_in : Inport  Unit=1
  mu ext : Subsystem  VariantControl=1
  mu ext dual : Subsystem  VariantControl=3
  mu int : Subsystem  VariantControl=0
  mu int dual : Subsystem  VariantControl=2
  mu_out : Outport  Unit=1  VectorParamsAs1DForOutWhenUnconnected=off

== system autolibshared/Vehicle Body 3DOF Single Track/front forces ==
  note: 1) Add Subsystem or Model blocks as valid variant choices.
      | 2) You cannot connect blocks at this level. At simulation, connectivity is automatically
      | determined, based on the active variant and port name matching.
  F_in : Inport  Unit=N
  ext : Subsystem  VariantControl=2
  ext dual : Subsystem  VariantControl=5
  ext long : Subsystem  VariantControl=1
  ext long dual : Subsystem  VariantControl=4
  int : Subsystem  VariantControl=0
  int dual : Subsystem  VariantControl=3
  F_out : Outport  Unit=N  VectorParamsAs1DForOutWhenUnconnected=off

== system autolibshared/Vehicle Body 3DOF Single Track/front steer ==
  note: 1) Add Subsystem or Model blocks as valid variant choices.
      | 2) You cannot connect blocks at this level. At simulation, connectivity is automatically
      | determined, based on the active variant and port name matching.
  delta_in : Inport  Unit=rad
  delta ext : Subsystem  VariantControl=1
  delta ext dual : Subsystem  VariantControl=3
  delta int : Subsystem  VariantControl=0
  delta int dual : Subsystem  VariantControl=2
  delta_out : Outport  Unit=rad  VectorParamsAs1DForOutWhenUnconnected=off

== system autolibshared/Vehicle Body 3DOF Single Track/sigma ==
  note: 1) Add Subsystem or Model blocks as valid variant choices.
      | 2) You cannot connect blocks at this level. At simulation, connectivity is automatically
      | determined, based on the active variant and port name matching.
  y : Inport
  no sigma : Subsystem  VariantControl=0
  no sigma dual : Subsystem  VariantControl=2
  sigma : Subsystem  VariantControl=1
  sigma dual : Subsystem  VariantControl=3
  alpha_f : Outport  VectorParamsAs1DForOutWhenUnconnected=off
  alpha_r : Outport  Port=2  VectorParamsAs1DForOutWhenUnconnected=off

== system autolibshared/Vehicle Body 3DOF Single Track/state ==
  note: 1) Add Subsystem or Model blocks as valid variant choices.
      | 2) You cannot connect blocks at this level. At simulation, connectivity is automatically
      | determined, based on the active variant and port name matching.
  xdot : Inport  Unit=m/s
  xddot_in : Inport  Port=2  PortDimensions=4
  extState : Inport  Port=3
  xdot ext : Subsystem  VariantControl=1
  xdot int : Subsystem  VariantControl=0
  xddot_out : Outport  VectorParamsAs1DForOutWhenUnconnected=off

== system autolibshared/Vehicle Body 3DOF Single Track/wind ==
  note: 1) Add Subsystem or Model blocks as valid variant choices.
      | 2) You cannot connect blocks at this level. At simulation, connectivity is automatically
      | determined, based on the active variant and port name matching.
  wind_in : Inport  Unit=m/s
  wind ext : Subsystem  VariantControl=1
  wind int : Subsystem  VariantControl=0
  wind_out : Outport  Unit=m/s  VectorParamsAs1DForOutWhenUnconnected=off

== system autolibshared/Drive Cycle Source/timing mode/Continuous ==
  1-D Lookup Table : Lookup_n-D  NumberOfTableDimensions=1  LookupTableObject=''  BreakpointsForDimension1=DriveCycle.Time  BeginIndexSearchUsingPreviousIndexResult=on  Table=DriveCycle.Data  ExtrapMethod=Clip  UseLastTableValue=on  InternalRulePriority=Speed  RndMeth=Simplest  InputSameDT=on
  1-D Lookup Table1 : Lookup_n-D  NumberOfTableDimensions=1  LookupTableObject=''  BreakpointsForDimension1=AccelCycle.Time  BeginIndexSearchUsingPreviousIndexResult=on  Table=AccelCycle.Data  ExtrapMethod=Clip  UseLastTableValue=on  InternalRulePriority=Speed  RndMeth=Simplest  InputSameDT=on
  1-D Lookup Table2 : Lookup_n-D  NumberOfTableDimensions=1  LookupTableObject=''  BreakpointsForDimension1=GearCycle.Time  BeginIndexSearchUsingPreviousIndexResult=on  Table=GearCycle.Data  InterpMethod=Flat  InternalRulePriority=Speed  RndMeth=Simplest  InputSameDT=on
  Add1 : Sum  Inputs=+-
  Clock : Clock
  Digital Clock : DigitalClock  SampleTime=min(0.5,(DriveCycle.Time(2)-DriveCycle.Time(1))./2)
  Hit Crossing : HitCross  HitCrossingOffset=min(0.5,(DriveCycle.Time(2)-DriveCycle.Time(1))./2)  HitCrossingDirection=falling  ShowOutputPort=off
  Math Function : Math  Operator=mod  SaturateOnIntegerOverflow=on
  Switch : Switch  Criteria=u2 > Threshold
  repeat : Constant  Value=cycleRepeat
  tFinal : Constant  Value=DriveCycle.Time(end)
  Spd : Outport  Unit=m/s  VectorParamsAs1DForOutWhenUnconnected=off
  Acc : Outport  Port=2  Unit=m/s/s  VectorParamsAs1DForOutWhenUnconnected=off
  Gear : Outport  Port=3  Unit=1  VectorParamsAs1DForOutWhenUnconnected=off
  wires:
  1-D Lookup Table2/1 -> Gear/1
  Switch/1 -> 1-D Lookup Table/1, 1-D Lookup Table1/1, 1-D Lookup Table2/1
  1-D Lookup Table1/1 -> Acc/1
  repeat/1 -> Switch/2
  Add1/1 -> Hit Crossing/1
  Digital Clock/1 -> Add1/2
  Clock/1 -> Math Function/1, Add1/1, Switch/3
  tFinal/1 -> Math Function/2
  Math Function/1 -> Switch/1
  1-D Lookup Table/1 -> Spd/1

== system autolibshared/Drive Cycle Source/timing mode/Discrete ==
  1-D Lookup Table : Lookup_n-D  NumberOfTableDimensions=1  LookupTableObject=''  BreakpointsForDimension1=DriveCycle.Time  BeginIndexSearchUsingPreviousIndexResult=on  Table=DriveCycle.Data  InternalRulePriority=Speed  RndMeth=Simplest  InputSameDT=on
  1-D Lookup Table1 : Lookup_n-D  NumberOfTableDimensions=1  LookupTableObject=''  BreakpointsForDimension1=AccelCycle.Time  BeginIndexSearchUsingPreviousIndexResult=on  Table=AccelCycle.Data  InternalRulePriority=Speed  RndMeth=Simplest  InputSameDT=on
  1-D Lookup Table2 : Lookup_n-D  NumberOfTableDimensions=1  LookupTableObject=''  BreakpointsForDimension1=GearCycle.Time  BeginIndexSearchUsingPreviousIndexResult=on  Table=GearCycle.Data  InterpMethod=Flat  InternalRulePriority=Speed  RndMeth=Simplest  InputSameDT=on
  Digital Clock : DigitalClock  SampleTime=dt
  Math Function : Math  Operator=mod  SaturateOnIntegerOverflow=on
  Switch : Switch  Criteria=u2 > Threshold
  repeat : Constant  Value=cycleRepeat
  tFinal : Constant  Value=DriveCycle.Time(end)
  Spd : Outport  Unit=m/s  VectorParamsAs1DForOutWhenUnconnected=off
  Acc : Outport  Port=2  Unit=m/s/s  VectorParamsAs1DForOutWhenUnconnected=off
  Gear : Outport  Port=3  Unit=1  VectorParamsAs1DForOutWhenUnconnected=off
  wires:
  1-D Lookup Table2/1 -> Gear/1
  1-D Lookup Table1/1 -> Acc/1
  Switch/1 -> 1-D Lookup Table/1, 1-D Lookup Table1/1, 1-D Lookup Table2/1
  repeat/1 -> Switch/2
  Math Function/1 -> Switch/1
  Digital Clock/1 -> Math Function/1, Switch/3
  tFinal/1 -> Math Function/2
  1-D Lookup Table/1 -> Spd/1

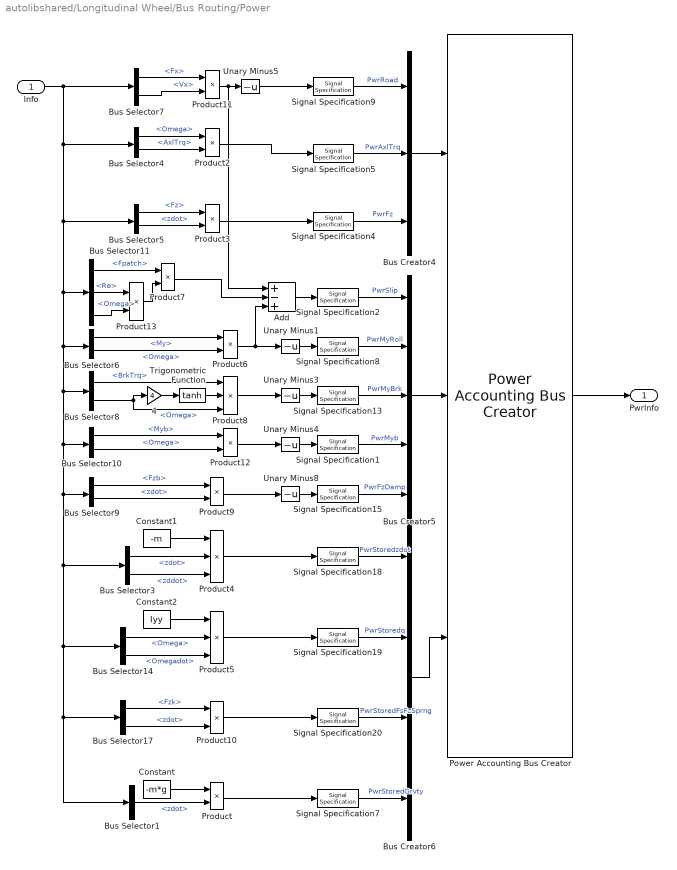
== system autolibshared/Longitudinal Wheel/Bus Routing/Power ==
  Info : Inport
  4 : Gain  Gain=4  SaturateOnIntegerOverflow=on  OutDataTypeStr=Inherit: Same as input  ParamDataTypeStr=Inherit: Same as input
  Add : Sum  Inputs=+-+
  Bus Creator4 : BusCreator  Inputs=3
  Bus Creator5 : BusCreator  Inputs=5
  Bus Creator6 : BusCreator  Inputs=4
  Bus Selector1 : BusSelector  OutputSignals=zdot
  Bus Selector10 : BusSelector  OutputSignals=Myb,Omega
  Bus Selector11 : BusSelector  OutputSignals=Fpatch,Re,Omega
  Bus Selector14 : BusSelector  OutputSignals=Omega,Omegadot
  Bus Selector17 : BusSelector  OutputSignals=Fzk,zdot
  Bus Selector3 : BusSelector  OutputSignals=zdot,zddot
  Bus Selector4 : BusSelector  OutputSignals=Omega,AxlTrq
  Bus Selector5 : BusSelector  OutputSignals=Fz,zdot
  Bus Selector6 : BusSelector  OutputSignals=My,Omega
  Bus Selector7 : BusSelector  OutputSignals=Fx,Vx
  Bus Selector8 : BusSelector  OutputSignals=BrkTrq,Omega
  Bus Selector9 : BusSelector  OutputSignals=Fzb,zdot
  Constant : Constant  Value=-m*g
  Constant1 : Constant  Value=-m
  Constant2 : Constant  Value=Iyy
  Power Accounting Bus Creator : autolibpowerinfoutils/Power Accounting Bus Creator  AssctBlkSelPopup=Parent reference block  RefBlkName='autolibshared/Longitudinal Wheel'  PwrTrnsfrdCheckBox=on  PwrNotTrnsfrdCheckBox=on  PwrStoredCheckBox=on  aMode=aMode
      settings: SourceProductName=Powertrain Blockset  SourceProductBaseCode=PW
  Product{,2..3,6..7,9..13} (10 alike) : Product
  Product4 : Product  Inputs=3
  Product5 : Product  Inputs=3
  Product8 : Product  Inputs=3
  Signal Specification{1..2,4..5,7..9,13,15,18..20} (12 alike) : SignalSpecification  Unit=W  Dimensions=1
  Trigonometric Function : Trigonometry  Operator=tanh
  Unary Minus{1,3..5,8} (5 alike) : UnaryMinus
  PwrInfo : Outport  VectorParamsAs1DForOutWhenUnconnected=off
  wires:
  Signal Specification8/1 -> Bus Creator5/2  "PwrMyRoll"
  Bus Creator6/1 -> Power Accounting Bus Creator/3
  Unary Minus1/1 -> Signal Specification8/1
  Signal Specification20/1 -> Bus Creator6/3  "PwrStoredFsFzSprng"
  Bus Selector14/1 -> Product5/2  "<Omega>"
  Bus Selector1/1 -> Product/2  "<zdot>"
  Signal Specification7/1 -> Bus Creator6/4  "PwrStoredGrvty"
  Bus Selector14/2 -> Product5/3  "<Omegadot>"
  Bus Creator5/1 -> Power Accounting Bus Creator/2
  Bus Creator4/1 -> Power Accounting Bus Creator/1
  Bus Selector3/1 -> Product4/2  "<zdot>"
  Signal Specification15/1 -> Bus Creator5/5  "PwrFzDamp"
  Signal Specification13/1 -> Bus Creator5/3  "PwrMyBrk"
  Constant1/1 -> Product4/1
  Signal Specification18/1 -> Bus Creator6/1  "PwrStoredzdot"
  Signal Specification19/1 -> Bus Creator6/2  "PwrStoredq"
  Bus Selector17/2 -> Product10/2  "<zdot>"
  Product10/1 -> Signal Specification20/1
  Product4/1 -> Signal Specification18/1
  Constant2/1 -> Product5/1
  Bus Selector6/1 -> Product6/1  "<My>"
  Constant/1 -> Product/1
  Bus Selector17/1 -> Product10/1  "<Fzk>"
  Signal Specification5/1 -> Bus Creator4/2  "PwrAxlTrq"
  Power Accounting Bus Creator/1 -> PwrInfo/1
  Signal Specification4/1 -> Bus Creator4/3  "PwrFz"
  Bus Selector3/2 -> Product4/3  "<zddot>"
  Bus Selector4/2 -> Product2/2  "<AxlTrq>"
  Bus Selector4/1 -> Product2/1  "<Omega>"
  Bus Selector5/1 -> Product3/1  "<Fz>"
  Bus Selector5/2 -> Product3/2  "<zdot>"
  Bus Selector6/2 -> Product6/2  "<Omega>"
  Bus Selector8/1 -> Product8/1  "<BrkTrq>"
  Trigonometric Function/1 -> Product8/2
  Bus Selector9/1 -> Product9/1  "<Fzb>"
  Bus Selector9/2 -> Product9/2  "<zdot>"
  Product9/1 -> Unary Minus8/1
  Bus Selector7/2 -> Product11/2  "<Vx>"
  Product11/1 -> Add/1, Unary Minus5/1
  Signal Specification2/1 -> Bus Creator5/1  "PwrSlip"
  Bus Selector10/2 -> Product12/2  "<Omega>"
  Bus Selector10/1 -> Product12/1  "<Myb>"
  Unary Minus3/1 -> Signal Specification13/1
  Product12/1 -> Unary Minus4/1
  Unary Minus4/1 -> Signal Specification1/1
  Product6/1 -> Add/3, Unary Minus1/1
  Product5/1 -> Signal Specification19/1
  Signal Specification9/1 -> Bus Creator4/1  "PwrRoad"
  Info/1 -> Bus Selector11/1, Bus Selector1/1, Bus Selector17/1, Bus Selector14/1, Bus Selector3/1, Bus Selector9/1, Bus Selector10/1, Bus Selector8/1, Bus Selector6/1, Bus Selector5/1, Bus Selector4/1, Bus Selector7/1
  4/1 -> Trigonometric Function/1
  Bus Selector8/2 -> Product8/3, 4/1  "<Omega>"
  Product8/1 -> Unary Minus3/1
  Product3/1 -> Signal Specification4/1
  Unary Minus8/1 -> Signal Specification15/1
  Product/1 -> Signal Specification7/1
  Signal Specification1/1 -> Bus Creator5/4  "PwrMyb"
  Bus Selector11/2 -> Product13/1  "<Re>"
  Bus Selector11/3 -> Product13/2  "<Omega>"
  Product13/1 -> Product7/2
  Add/1 -> Signal Specification2/1
  Bus Selector7/1 -> Product11/1  "<Fx>"
  Bus Selector11/1 -> Product7/1  "<Fpatch>"
  Product7/1 -> Add/2
  Unary Minus5/1 -> Signal Specification9/1
  Product2/1 -> Signal Specification5/1

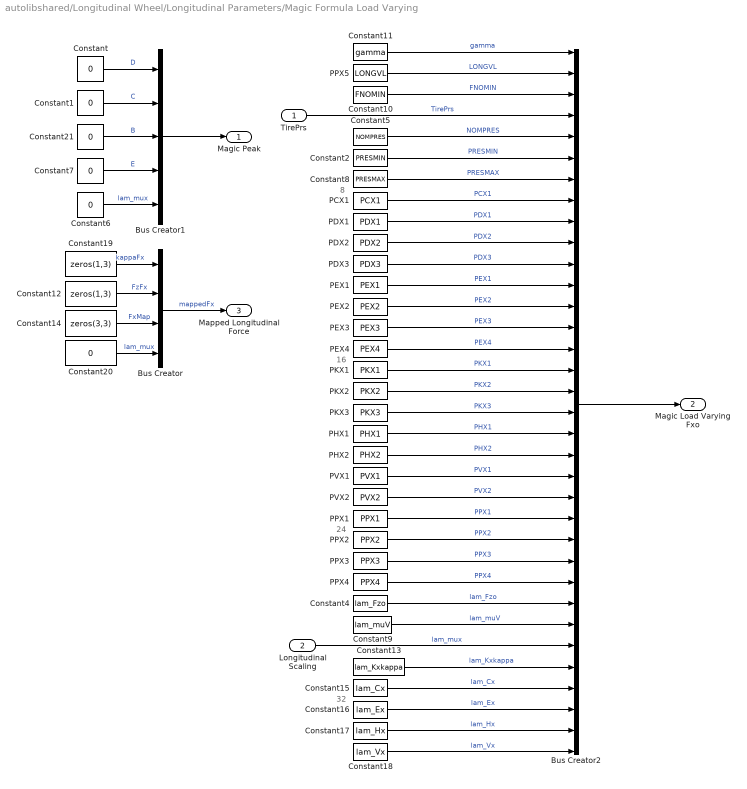
== system autolibshared/Longitudinal Wheel/Longitudinal Parameters/Magic Formula Load Varying ==
  note: 16
  note: 8
  note: 24
  note: 32
  TirePrs : Inport
  Longitudinal Scaling : Inport  Port=2
  Bus Creator : BusCreator  Inputs=4
  Bus Creator1 : BusCreator  Inputs=5
  Bus Creator2 : BusCreator  Inputs=34
  Constant{,1,6..7,20..21} (6 alike) : Constant  Value=0
  Constant10 : Constant  Value=FNOMIN
  Constant11 : Constant  Value=gamma
  Constant12 : Constant  Value=zeros(1,3)
  Constant13 : Constant  Value=lam_Kxkappa
  Constant14 : Constant  Value=zeros(3,3)
  Constant15 : Constant  Value=lam_Cx
  Constant16 : Constant  Value=lam_Ex
  Constant17 : Constant  Value=lam_Hx
  Constant18 : Constant  Value=lam_Vx
  Constant19 : Constant  Value=zeros(1,3)
  Constant2 : Constant  Value=PRESMIN
  Constant4 : Constant  Value=lam_Fzo
  Constant5 : Constant  Value=NOMPRES
  Constant8 : Constant  Value=PRESMAX
  Constant9 : Constant  Value=lam_muV
  PCX1 : Constant  Value=PCX1
  PDX1 : Constant  Value=PDX1
  PDX2 : Constant  Value=PDX2
  PDX3 : Constant  Value=PDX3
  PEX1 : Constant  Value=PEX1
  PEX2 : Constant  Value=PEX2
  PEX3 : Constant  Value=PEX3
  PEX4 : Constant  Value=PEX4
  PHX1 : Constant  Value=PHX1
  PHX2 : Constant  Value=PHX2
  PKX1 : Constant  Value=PKX1
  PKX2 : Constant  Value=PKX2
  PKX3 : Constant  Value=PKX3
  PPX1 : Constant  Value=PPX1
  PPX2 : Constant  Value=PPX2
  PPX3 : Constant  Value=PPX3
  PPX4 : Constant  Value=PPX4
  PPX5 : Constant  Value=LONGVL
  PVX1 : Constant  Value=PVX1
  PVX2 : Constant  Value=PVX2
  Magic Peak : Outport  VectorParamsAs1DForOutWhenUnconnected=off
  Magic Load Varying Fxo : Outport  Port=2  VectorParamsAs1DForOutWhenUnconnected=off
  Mapped Longitudinal Force : Outport  Port=3  VectorParamsAs1DForOutWhenUnconnected=off
  wires:
  Longitudinal Scaling/1 -> Bus Creator2/29  "lam_mux"
  Constant7/1 -> Bus Creator1/4  "E"
  Constant1/1 -> Bus Creator1/2  "C"
  Constant/1 -> Bus Creator1/1  "D"
  Bus Creator1/1 -> Magic Peak/1
  Constant21/1 -> Bus Creator1/3  "B"
  Constant6/1 -> Bus Creator1/5  "lam_mux"
  Constant14/1 -> Bus Creator/3  "FxMap"
  Constant12/1 -> Bus Creator/2  "FzFx"
  Bus Creator/1 -> Mapped Longitudinal Force/1  "mappedFx"
  Constant19/1 -> Bus Creator/1  "kappaFx"
  Constant20/1 -> Bus Creator/4  "lam_mux"
  Constant18/1 -> Bus Creator2/34  "lam_Vx"
  Constant17/1 -> Bus Creator2/33  "lam_Hx"
  Constant16/1 -> Bus Creator2/32  "lam_Ex"
  Constant15/1 -> Bus Creator2/31  "lam_Cx"
  Constant13/1 -> Bus Creator2/30  "lam_Kxkappa"
  Constant9/1 -> Bus Creator2/28  "lam_muV"
  Constant4/1 -> Bus Creator2/27  "lam_Fzo"
  Constant8/1 -> Bus Creator2/7  "PRESMAX"
  Constant2/1 -> Bus Creator2/6  "PRESMIN"
  Constant5/1 -> Bus Creator2/5  "NOMPRES"
  Bus Creator2/1 -> Magic Load Varying Fxo/1
  PPX5/1 -> Bus Creator2/2  "LONGVL"
  PPX4/1 -> Bus Creator2/26  "PPX4"
  PPX3/1 -> Bus Creator2/25  "PPX3"
  PPX2/1 -> Bus Creator2/24  "PPX2"
  PPX1/1 -> Bus Creator2/23  "PPX1"
  PVX2/1 -> Bus Creator2/22  "PVX2"
  PVX1/1 -> Bus Creator2/21  "PVX1"
  PHX2/1 -> Bus Creator2/20  "PHX2"
  PHX1/1 -> Bus Creator2/19  "PHX1"
  PKX3/1 -> Bus Creator2/18  "PKX3"
  PKX2/1 -> Bus Creator2/17  "PKX2"
  PKX1/1 -> Bus Creator2/16  "PKX1"
  PEX4/1 -> Bus Creator2/15  "PEX4"
  PEX3/1 -> Bus Creator2/14  "PEX3"
  PEX2/1 -> Bus Creator2/13  "PEX2"
  PEX1/1 -> Bus Creator2/12  "PEX1"
  PDX3/1 -> Bus Creator2/11  "PDX3"
  PDX2/1 -> Bus Creator2/10  "PDX2"
  PDX1/1 -> Bus Creator2/9  "PDX1"
  PCX1/1 -> Bus Creator2/8  "PCX1"
  Constant11/1 -> Bus Creator2/1  "gamma"
  Constant10/1 -> Bus Creator2/3  "FNOMIN"
  TirePrs/1 -> Bus Creator2/4  "TirePrs"
